simulink model "lab8"  (Simulink 8.5)
settings: Solver=ode45  StartTime=0.0  StopTime=10000000  RelTol=1e-3
settings Model: Creator=Meteo  LastModifiedBy=Meteo
settings DataIOCC: SignalLoggingSaveFormat=Dataset
settings OptimizationCC: ExpressionDepthLimit=128
settings DebuggingCC: UnderspecifiedInitializationDetection=Simplified  MergeDetectMultiDrivingBlocksExec=error  FcnCallInpInsideContextMsg=EnableAllAsError  StateNameClashWarn=none
settings GRTTargetCC: CombineOutputUpdateFcns=on  GRTInterface=off

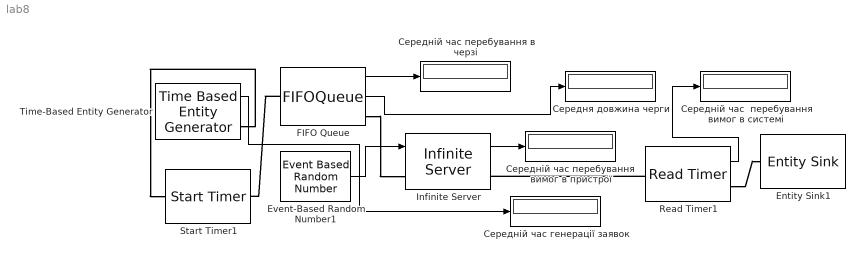
== system lab8 ==
  Entity Sink1 : EntitySink
  Event-Based Random Number1 : EventBasedRandomNumber  meanExp=17  Seed=61357
  FIFO Queue : FIFOQueue  StatAverageWait=on  StatAverageQueueLength=on
      settings: OutputPortMap=o2,o3
  Infinite Server : InfiniteServer  ServiceTimeFrom=Signal port t  StatAverageWait=on
      settings: OutputPortMap=o4
  Read Timer1 : ReadTimer  StatAverageTimeElapsed=on
      settings: OutputPortMap=o3
  Start Timer1 : StartTimer
  Time-Based Entity Generator : TimeBasedEntityGenerator  Distribution=Exponential  Period=27  InitialSeed=64574  Mean=27  StatAverageIntergenerationTime=on
      settings: OutputPortMap=o2
  Середня довжина черги : Display
  Середній час  перебування вимог в системі : Display
  Середній час генерації заявок : Display
  "Середній час перебування  вимог в пристрої " : Display
  Середній час перебування в черзі : Display
  wires:
  Infinite Server/1 -> "Середній час перебування  вимог в пристрої "/1
  Read Timer1/1 -> Середній час  перебування вимог в системі/1
  FIFO Queue/2 -> Середня довжина черги/1
  FIFO Queue/1 -> Середній час перебування в черзі/1
  Event-Based Random Number1/1 -> Infinite Server/1
  Time-Based Entity Generator/1 -> Середній час генерації заявок/1
  connections:
  Read Timer1/LConn1 -- Infinite Server/RConn1
  FIFO Queue/RConn1 -- Infinite Server/LConn1
  FIFO Queue/LConn1 -- Start Timer1/RConn1
  Read Timer1/RConn1 -- Entity Sink1/LConn1
  Time-Based Entity Generator/RConn1 -- Start Timer1/LConn1
